simulink model "buoy_detector"  (Simulink 7.6)
settings: Solver=FixedStepDiscrete  StartTime=0.0  StopTime=0  FixedStep=1/30  RelTol=1e-3
values from neighbouring files (symbols this model uses):
  Buoy_Count_Max = 50    [VisionConstants.m]
  Buoy_Count_Min = 3    [VisionConstants.m]
  Buoy_Max_Eccentricity = 1.2    [VisionConstants.m]
  Buoy_Max_Extent = 0.9    [VisionConstants.m]
  Buoy_Min_Eccentricity = 0    [VisionConstants.m]
  Buoy_Min_Extent = 0.1    [VisionConstants.m]
  Iter_Segment_Thresh = 60    [VisionConstants.m]
undefined symbols (not defined in the file or in its folder): Rec, SDTV
libraries: vipgeotforms x3, vipconversions x1
settings Model: Creator=auvt  LastModifiedBy=Administrator
settings RTWCC: TargetLang=C++

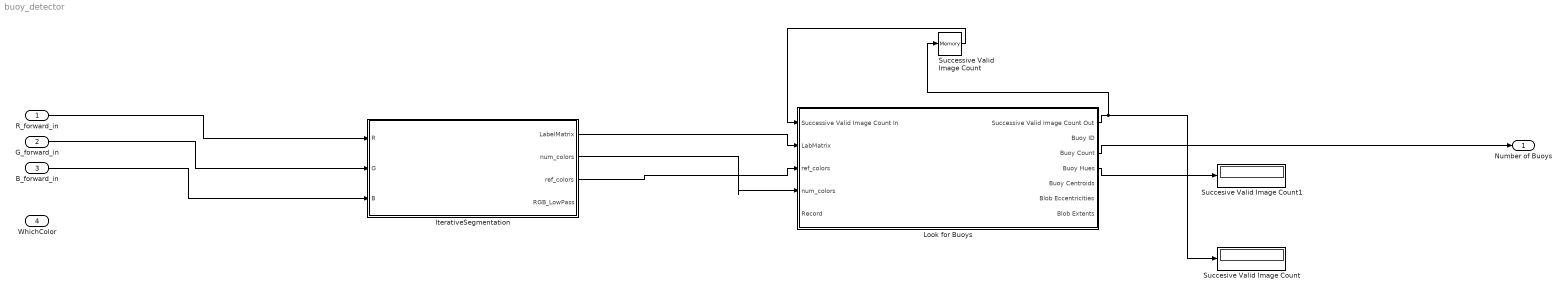
== system buoy_detector ==
  R_forward_in : Inport  PortDimensions=Forward_Camera_Dimensions
  G_forward_in : Inport  Port=2  PortDimensions=Forward_Camera_Dimensions
  B_forward_in : Inport  Port=3  PortDimensions=Forward_Camera_Dimensions
  WhichColor : Inport  Port=4
  IterativeSegmentation : Subsystem
      settings: UndoDeleteFcn=Stateflow.SLINSF.SimulinkMan.restorePreDeleteFcn  PreDeleteFcn=Stateflow.SLINSF.SimulinkMan.removePreDeleteFcn
  Look for Buoys : Subsystem
      settings: UndoDeleteFcn=Stateflow.SLINSF.SimulinkMan.restorePreDeleteFcn  PreDeleteFcn=Stateflow.SLINSF.SimulinkMan.removePreDeleteFcn
  Succesive Valid Image Count : Display
  Succesive Valid Image Count1 : Display
  Successive Valid Image Count : Memory
  Number of Buoys : Outport
  wires:
  IterativeSegmentation/1(LabelMatrix) -> Look for Buoys/2(LabMatrix)
  IterativeSegmentation/3(ref_colors) -> Look for Buoys/3(ref_colors)
  IterativeSegmentation/2(num_colors) -> Look for Buoys/4(num_colors)
  Look for Buoys/3(Buoy Count) -> Number of Buoys/1
  Look for Buoys/1(Successive Valid Image Count Out) -> Succesive Valid Image Count/1, Successive Valid Image Count/1
  Look for Buoys/4(Buoy Hues) -> Succesive Valid Image Count1/1
  Successive Valid Image Count/1 -> Look for Buoys/1(Successive Valid Image Count In)
  R_forward_in/1 -> IterativeSegmentation/1(R)
  G_forward_in/1 -> IterativeSegmentation/2(G)
  B_forward_in/1 -> IterativeSegmentation/3(B)

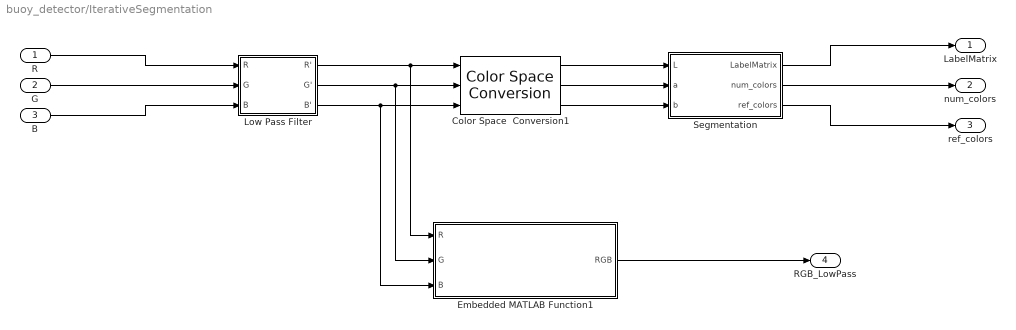
== system buoy_detector/IterativeSegmentation ==
  R : Inport
  G : Inport  Port=2
  B : Inport  Port=3
  Color Space  Conversion1 : vipconversions/Color Space  Conversion  conversion=Obsolete  conversionActive=sR'G'B' to L*a*b*  wp_str=D50  rec=Rec. 601 (SDTV)  sys=1125/60/2:1  imagePorts=Separate color signals
  Embedded MATLAB Function1 : Stateflow chart  TreatAsAtomicUnit=on
  Low Pass Filter : Subsystem
  Segmentation : Subsystem
  LabelMatrix : Outport
  num_colors : Outport  Port=2
  ref_colors : Outport  Port=3
  RGB_LowPass : Outport  Port=4
  wires:
  Segmentation/3(ref_colors) -> ref_colors/1
  Segmentation/2(num_colors) -> num_colors/1
  Segmentation/1(LabelMatrix) -> LabelMatrix/1
  Low Pass Filter/3(B') -> Color Space  Conversion1/3, Embedded MATLAB Function1/3(B)
  Low Pass Filter/2(G') -> Color Space  Conversion1/2, Embedded MATLAB Function1/2(G)
  Low Pass Filter/1(R') -> Color Space  Conversion1/1, Embedded MATLAB Function1/1(R)
  Color Space  Conversion1/3 -> Segmentation/3(b)
  Color Space  Conversion1/2 -> Segmentation/2(a)
  Color Space  Conversion1/1 -> Segmentation/1(L)
  Embedded MATLAB Function1/1(RGB) -> RGB_LowPass/1
  R/1 -> Low Pass Filter/1(R)
  G/1 -> Low Pass Filter/2(G)
  B/1 -> Low Pass Filter/3(B)

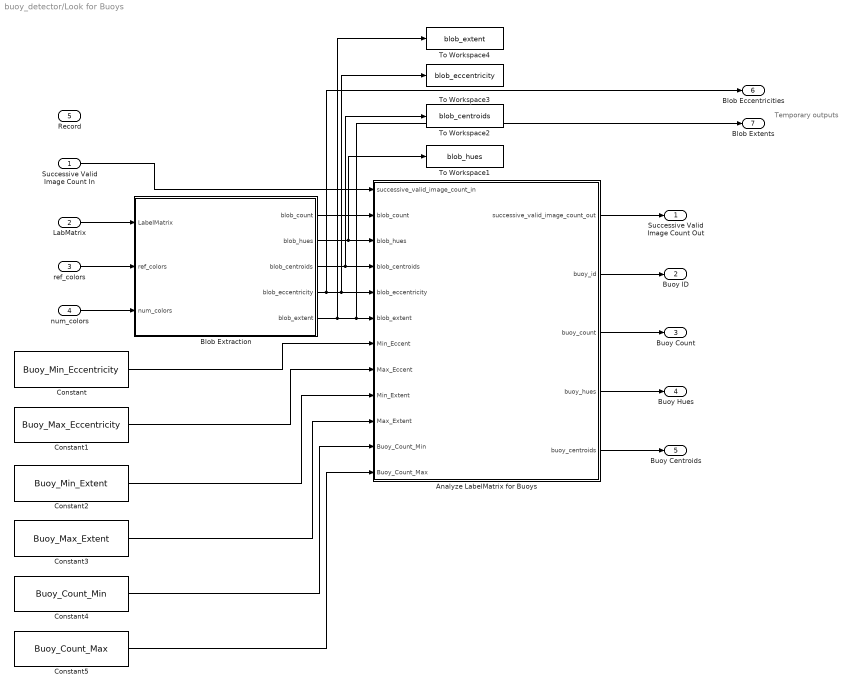
== system buoy_detector/Look for Buoys ==
  note: Temporary outputs
  Successive Valid Image Count In : Inport
  LabMatrix : Inport  Port=2
  ref_colors : Inport  Port=3
  num_colors : Inport  Port=4
  Record : Inport  Port=5
  Analyze LabelMatrix for Buoys : Stateflow chart  TreatAsAtomicUnit=on
  Blob Extraction : Stateflow chart  TreatAsAtomicUnit=on
  Constant : Constant  Value=Buoy_Min_Eccentricity  SampleTime=-1
  Constant1 : Constant  Value=Buoy_Max_Eccentricity  SampleTime=-1
  Constant2 : Constant  Value=Buoy_Min_Extent  SampleTime=-1
  Constant3 : Constant  Value=Buoy_Max_Extent  SampleTime=-1
  Constant4 : Constant  Value=Buoy_Count_Min  SampleTime=-1
  Constant5 : Constant  Value=Buoy_Count_Max  SampleTime=-1
  To Workspace1 : ToWorkspace  VariableName=blob_hues  SampleTime=-1  SaveFormat=Array
  To Workspace2 : ToWorkspace  VariableName=blob_centroids  SampleTime=-1  SaveFormat=Array
  To Workspace3 : ToWorkspace  VariableName=blob_eccentricity  SampleTime=-1  SaveFormat=Array
  To Workspace4 : ToWorkspace  VariableName=blob_extent  SampleTime=-1  SaveFormat=Array
  Successive Valid Image Count Out : Outport
  Buoy ID : Outport  Port=2
  Buoy Count : Outport  Port=3
  Buoy Hues : Outport  Port=4
  Buoy Centroids : Outport  Port=5
  Blob Eccentricities : Outport  Port=6
  Blob Extents : Outport  Port=7
  wires:
  num_colors/1 -> Blob Extraction/3(num_colors)
  LabMatrix/1 -> Blob Extraction/1(LabelMatrix)
  Blob Extraction/1(blob_count) -> Analyze LabelMatrix for Buoys/2(blob_count)
  Blob Extraction/2(blob_hues) -> Analyze LabelMatrix for Buoys/3(blob_hues), To Workspace1/1
  Blob Extraction/3(blob_centroids) -> Analyze LabelMatrix for Buoys/4(blob_centroids), To Workspace2/1
  Blob Extraction/4(blob_eccentricity) -> Analyze LabelMatrix for Buoys/5(blob_eccentricity), To Workspace3/1, Blob Eccentricities/1
  Blob Extraction/5(blob_extent) -> To Workspace4/1, Analyze LabelMatrix for Buoys/6(blob_extent), Blob Extents/1
  Constant/1 -> Analyze LabelMatrix for Buoys/7(Min_Eccent)
  Constant1/1 -> Analyze LabelMatrix for Buoys/8(Max_Eccent)
  Constant2/1 -> Analyze LabelMatrix for Buoys/9(Min_Extent)
  Constant3/1 -> Analyze LabelMatrix for Buoys/10(Max_Extent)
  Constant4/1 -> Analyze LabelMatrix for Buoys/11(Buoy_Count_Min)
  Constant5/1 -> Analyze LabelMatrix for Buoys/12(Buoy_Count_Max)
  Analyze LabelMatrix for Buoys/1(successive_valid_image_count_out) -> Successive Valid Image Count Out/1
  Analyze LabelMatrix for Buoys/3(buoy_count) -> Buoy Count/1
  Analyze LabelMatrix for Buoys/4(buoy_hues) -> Buoy Hues/1
  Analyze LabelMatrix for Buoys/5(buoy_centroids) -> Buoy Centroids/1
  Successive Valid Image Count In/1 -> Analyze LabelMatrix for Buoys/1(successive_valid_image_count_in)
  ref_colors/1 -> Blob Extraction/2(ref_colors)
  Analyze LabelMatrix for Buoys/2(buoy_id) -> Buoy ID/1

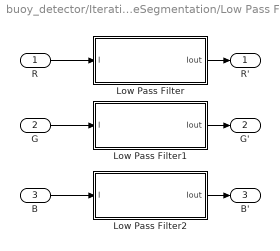
== system buoy_detector/IterativeSegmentation/Low Pass Filter ==
  R : Inport
  G : Inport  Port=2
  B : Inport  Port=3
  Low Pass Filter : Stateflow chart  TreatAsAtomicUnit=on
  Low Pass Filter1 : Stateflow chart  TreatAsAtomicUnit=on
  Low Pass Filter2 : Stateflow chart  TreatAsAtomicUnit=on
  R' : Outport
  G' : Outport  Port=2
  B' : Outport  Port=3
  wires:
  Low Pass Filter/1(Iout) -> R'/1
  Low Pass Filter2/1(Iout) -> B'/1
  Low Pass Filter1/1(Iout) -> G'/1
  B/1 -> Low Pass Filter2/1(I)
  G/1 -> Low Pass Filter1/1(I)
  R/1 -> Low Pass Filter/1(I)

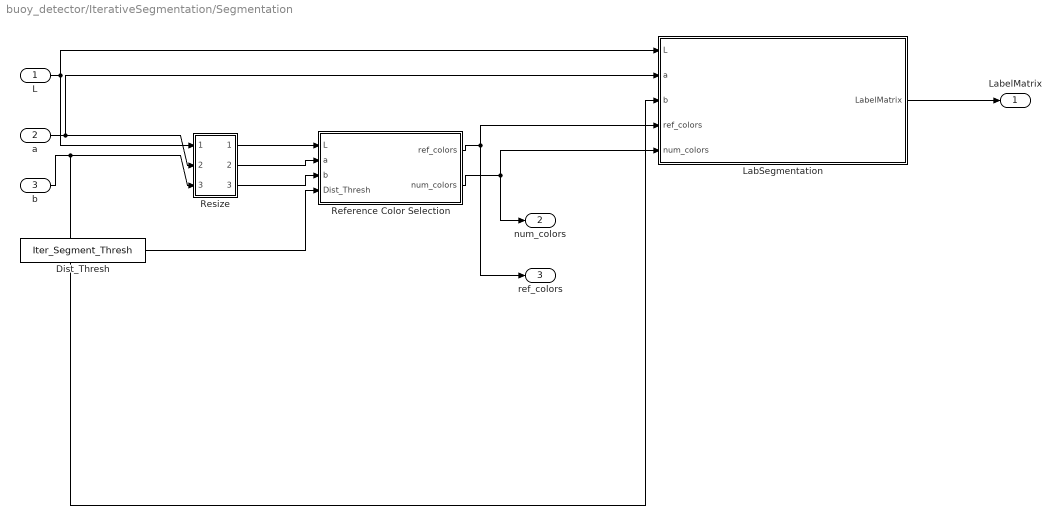
== system buoy_detector/IterativeSegmentation/Segmentation ==
  L : Inport
  a : Inport  Port=2
  b : Inport  Port=3
  Dist_Thresh : Constant  Value=Iter_Segment_Thresh  SampleTime=-1
  LabSegmentation : Stateflow chart  TreatAsAtomicUnit=on
  Reference Color Selection : Stateflow chart  TreatAsAtomicUnit=on
  Resize : Subsystem
  LabelMatrix : Outport
  num_colors : Outport  Port=2
  ref_colors : Outport  Port=3
  wires:
  Dist_Thresh/1 -> Reference Color Selection/4(Dist_Thresh)
  LabSegmentation/1(LabelMatrix) -> LabelMatrix/1
  Reference Color Selection/2(num_colors) -> LabSegmentation/5(num_colors), num_colors/1
  Reference Color Selection/1(ref_colors) -> ref_colors/1, LabSegmentation/4(ref_colors)
  Resize/3(Out3) -> Reference Color Selection/3(b)
  Resize/2(Out2) -> Reference Color Selection/2(a)
  Resize/1(Out1) -> Reference Color Selection/1(L)
  b/1 -> LabSegmentation/3(b), Resize/3(In3)
  a/1 -> LabSegmentation/2(a), Resize/2(In2)
  L/1 -> LabSegmentation/1(L), Resize/1(In1)

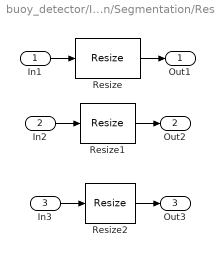
== system buoy_detector/IterativeSegmentation/Segmentation/Resize ==
  In1 : Inport
  In2 : Inport  Port=2
  In3 : Inport  Port=3
  Resize : vipgeotforms/Resize  DialogController=vipDDGCreate  DialogControllerArgs=DataTag0  specify=Number of output rows and columns  rfactor=[]  outCols=25  outRows=25  outRowsCols=[60 80]  interp_method=Bilinear  antialias=on  useROI=off  roiFlag=off  prodOutputMode=Binary point scaling  prodOutputWordLength=32  prodOutputFracLength=10  roundingMode=Nearest  overflowMode=on
  Resize1 : vipgeotforms/Resize  DialogController=vipDDGCreate  DialogControllerArgs=DataTag1  specify=Number of output rows and columns  rfactor=[200 150]  outCols=25  outRows=25  outRowsCols=[60 80]  interp_method=Bilinear  antialias=on  useROI=off  roiFlag=off  prodOutputMode=Binary point scaling  prodOutputWordLength=32  prodOutputFracLength=10  roundingMode=Nearest  overflowMode=on
  Resize2 : vipgeotforms/Resize  DialogController=vipDDGCreate  DialogControllerArgs=DataTag2  specify=Number of output rows and columns  rfactor=[200 150]  outCols=25  outRows=25  outRowsCols=[60 80]  interp_method=Bilinear  antialias=on  useROI=off  roiFlag=off  prodOutputMode=Binary point scaling  prodOutputWordLength=32  prodOutputFracLength=10  roundingMode=Nearest  overflowMode=on
  Out1 : Outport
  Out2 : Outport  Port=2
  Out3 : Outport  Port=3
  wires:
  Resize2/1 -> Out3/1
  In3/1 -> Resize2/1
  Resize1/1 -> Out2/1
  In2/1 -> Resize1/1
  Resize/1 -> Out1/1
  In1/1 -> Resize/1

== matlab function Look for Buoys/Blob Extraction ==
  data: blob_count output double; blob_hues output double; blob_centroids output double; LabelMatrix input double; ref_colors input double; blob_eccentricity output double; num_colors input double; blob_extent output double
function [blob_count, blob_hues, blob_centroids, blob_eccentricity, blob_extent] = GetBlobInfo(LabelMatrix, ref_colors, num_colors)
% This function will determine the characteristics of the blobs in an image
% given a label matrix defining the different binary images contained in a
% that label matrix
%
% Input
%   LabelMatrix = 2-D matrix of integer values, each of which represents a
%     color; location in matrix corresponds to pixel location in image
%   num_colors = integer number of colors present in LabelMatrix
%
% Output
%   blob_count = integer number of blobs in image
%   blob_hues = Nx1 vector of hues of blobs in image
%   blob_centroids = Nx2 matrix of x-y pairs of blob centroid locations
%   blob_eccentricity = Nx1 vector of blob eccentricites
%   blob_extent = Nx1 vector of blob extents


% Initialize
[rows, cols] = size(LabelMatrix);
LogicMatrix = false(rows,cols);

max_num_blobs = 50;
min_blob_area = 5;

blob_hues = double(zeros(max_num_blobs,3));
blob_centroids = double(zeros(max_num_blobs,2));
blob_eccentricity = double(zeros(max_num_blobs,1));
blob_extent = double(zeros(max_num_blobs,1));

blob_count = double(0);%uint8(0);

% Input hblob, a matrix containing [Area, blob_centroids, Eccentricity] for each
% identified blob
persistent hblob
if isempty(hblob)
    hblob = video.BlobAnalysis('AreaOutputPort',false,'BoundingBoxOutputPort',false,...
        'CentroidOutputPort',true,'EccentricityOutputPort',true,'ExtentOutputPort',true,...
        'NumBlobsOutputPort',true,'MinimumBlobAreaSource','Property',...
        'MinimumBlobArea', min_blob_area);
end

%% Calculate geometric information about the blobs
%
% LogicMatrix is a binary version of LabelMatrix, with ones at all
%   locations for which color values are k, and zeros everywhere else
for k = 1:num_colors
    for i = 1:rows
        for j = 1:cols
            if(LabelMatrix(i,j) ~= k)
                LogicMatrix(i,j) = false;
            else
                LogicMatrix(i,j) = true;
            end
        end
    end
    [TCentroid,TEccent,TExtent,TNumBlobs] = step(hblob,LogicMatrix);
    
    if(blob_count+TNumBlobs < max_num_blobs)
        for i = 1:TNumBlobs
            
            blob_centroids(blob_count+i,1) = TCentroid(1,i);
            blob_centroids(blob_count+i,2) = TCentroid(2,i);
            blob_eccentricity(blob_count+i) = TEccent(i);
            blob_extent(blob_count+i) = TExtent(i);
            
            ii = round(blob_centroids(blob_count+i,1));
            jj = round(blob_centroids(blob_count+i,2));
            blob_hues(blob_count+i,1) = ref_colors( LabelMatrix(ii,jj) );
            
        end
        blob_count = blob_count + 1;%TNumBlobs;
    end
end

return

== matlab function Look for Buoys/Analyze LabelMatrix for Buoys ==
  data: successive_valid_image_count_in input double; successive_valid_image_count_out output double; buoy_id output double; blob_count input double; blob_hues input double; blob_centroids input double; buoy_count output double; buoy_hues output double; buoy_centroids output double; blob_eccentricity input double; blob_extent input double; Min_Eccent input double; Max_Eccent input double; Min_Extent input double; Max_Extent input double; Buoy_Count_Min input double; Buoy_Count_Max input double
function [successive_valid_image_count_out, buoy_id, buoy_count, buoy_hues, buoy_centroids] = Buoy_Extraction(successive_valid_image_count_in, blob_count, blob_hues, blob_centroids, blob_eccentricity, blob_extent, Min_Eccent, Max_Eccent, Min_Extent, Max_Extent, Buoy_Count_Min, Buoy_Count_Max)
% This function takes in vectors representing blobs present in the image,
%   and returns information about how many and what kind of buoys are
%   present.
%
% Input
%   blob_count = integer number of blobs in image
%   blob_hues = Nx1 vector of hues of blobs in image
%   blob_centroids = Nx2 matrix of x-y pairs of blob centroid locations
%   blob_eccentricity = Nx1 vector of blob eccentricites
%   blob_extent = Nx1 vector of blob extents
%
%   Buoy_Count_Min = integer; minimum number of buoys searched for in an
%     image (mission/controls needs requires this option)
%   Buoy_Count_Max = maximum number of buoys allowed per image; arbitrary
%     limit
%   Min_Hue,Max_Hue = Nx1 limits on valid buoy hues; hue is between 0 and 1
%   Min_Eccent,Max_Eccent = scalar limits on buoy eccentricity
%   Min_Extent,Max_Extent = scalar limits on buoy extent
%
% Output
%   successive_valid_image_count = integer value of the number of times an
%     image with more than Min_Num_Buoys is processed; persistant between
%     function calls, so that the number of successive images containing
%     at least Min_Num_Buoys buoys is tracked
%   buoy_count = integer number of buoys in image
%   buoy_hues = Nx1 vector of buoy colors
%   buoy_centroids = Nx2 matrix of x-y pairs of buoy centroid locations


% Initialize
%persistent successive_valid_image_count;
buoy_count = double(0);

%debug
%successive_valid_image_count = 0;
Buoy_Count_Max = 50;


%/debug
buoy_hues = double(zeros(Buoy_Count_Max,1));
buoy_centroids = double(-500.*ones(Buoy_Count_Max,2));  % Initialize to points clearly not located in image

buoy_id = double(-1.*ones(Buoy_Count_Max,1));
Buoy_Hue_HalfRange = 10;
Buoy1_Hue = 30;
Buoy2_Hue = 80;
Buoy3_Hue = 15;

% Loop through blobs, and analyze and extract buoy information
for i = 1:blob_count
    
    % Convert Lab to XYZ
%    R = buoy_hues(i);
%    G = buoy_hues(i);
%    B = buoy_hues(i);
    
    L = blob_hues(:,1); %refcolors(LabelMatrix(1,1,1));
    a = blob_hues(:,2);
    b = blob_hues(:,3);
    
    var_Y = L./10;
    var_X = ( a./17.5 ).*( L./10 );
    var_Z = ( b./7 ).*( L./10 );
    
    Y = var_Y.^2;
    X = ( var_X + Y )./1.02;
    Z = -( var_Z - Y )./0.847;
    
    % Convert XYZ to RGB
    var_X = X./100;        %X from 0 to  95.047      (Observer = 2 degrees, Illuminant = D65)
    var_Y = Y./100;        %Y from 0 to 100.000
    var_Z = Z./100;        %Z from 0 to 108.883
    
    var_R = var_X.*3.2406 + var_Y.*(-1.5372) + var_Z.* -0.4986;
    var_G = var_X .* -0.9689 + var_Y .*  1.8758 + var_Z.*  0.0415;
    var_B = var_X .*  0.0557 + var_Y .* -0.2040 + var_Z .*  1.0570;
    
    var_R = ( var_R > 0.0031308 ).*( 1.055.*( var_R.^( 1./2.4 ) ) - 0.055 ) + ( var_R <= 0.0031308 ).*(12.92.*var_R);
    var_G = ( var_G > 0.0031308 ).*( 1.055.*( var_G.^( 1./2.4 ) ) - 0.055 ) + ( var_G <= 0.0031308 ).*( var_G <= 12.92.*var_G );
    var_B = ( var_B > 0.0031308 ).*( 1.055 .* ( var_B .^ ( 1 ./ 2.4 ) ) - 0.055 ) + ( var_B <= 0.0031308 ).*( 12.92 .* var_B );
    
    R = var_R .* 255;
    G = var_G .* 255;
    B = var_B .* 255;
    
    % Convert RGB to HSV
    var_R = ( R ./ 255 );  % RGB from 0 to 255
    var_G = ( G ./ 255 );
    var_B = ( B ./ 255 );
    
    var_Min = min( [var_R, var_G, var_B], [], 2 );  % Min. value of RGB
    var_Max = max( [var_R, var_G, var_B], [], 2 );  % Max. value of RGB
    del_Max = var_Max - var_Min;  % Delta RGB value
    
    V = var_Max;
    
%    H = (del_Max != 0).*(  );
%    S = (del_Max != 0).*( del_Max./var_Max );
    if ( max(abs(del_Max == 0)) );  % This is a gray, no chroma...
        H = zeros(size(var_R));  % HSV results from 0 to 1
        S = zeros(size(var_R));
    else  % Chromatic data...
        
        S = del_Max ./ var_Max;
        
        del_R = ( ( ( var_Max - var_R ) ./ 6 ) + ( del_Max ./ 2 ) ) ./ del_Max;
        del_G = ( ( ( var_Max - var_G ) ./ 6 ) + ( del_Max ./ 2 ) ) ./ del_Max;
        del_B = ( ( ( var_Max - var_B ) ./ 6 ) + ( del_Max ./ 2 ) ) ./ del_Max;
        
        
        H = ( var_R == var_Max ).*( del_B - del_G ) + ( var_G == var_Max ).*( ( 1 ./ 3 ) + del_R - del_B ) + ( var_B == var_Max ).*( ( 2 ./ 3 ) + del_G - del_R );
        H = ( H < 0 ).*( H + 1 ) + ( H > 1 ).*( H - 1 );
        
        
%{        
        if( var_R == var_Max )
            H = del_B - del_G;
        elseif( var_G == var_Max )
            H = ( 1 ./ 3 ) + del_R - del_B;
        elseif( var_B == var_Max )
            H = ( 2 ./ 3 ) + del_G - del_R;
        else
            H = 0;
        end
        
        if( H < 0 )
            H = H + 1;
        end
        if( H > 1 )
            H = H - 1;
        end
%}        
    end
    
    
    
    
    
    
    
    
    
    % Store buoy information if blob conditions are met
    %   Conditions: 1) Blob eccentricity is within specified range
    %               2) Blob extent is within specified range
    %               3) Blob hue is within specified range for several buoy
    %                 types
    if( (blob_eccentricity(i)>=Min_Eccent) && (blob_eccentricity(i)<=Max_Eccent) && (blob_extent(i)>=Min_Extent) && (blob_extent(i)<=Max_Extent) )
        
        %if( (blob_hues(i)>=Buoy1_Hue-Buoy_Hue_HalfRange) && (blob_hues(i)<=Buoy1_Hue+Buoy_Hue_HalfRange) )
            buoy_count = buoy_count + 1;
            buoy_hues(buoy_count) = blob_hues(i);
            buoy_id(buoy_count) = 1;
            buoy_centroids(buoy_count,1) = blob_centroids(i,1);
            buoy_centroids(buoy_count,2) = blob_centroids(i,2);
        %end
        if( (blob_hues(i)>=Buoy2_Hue-Buoy_Hue_HalfRange) && (blob_hues(i)<=Buoy2_Hue+Buoy_Hue_HalfRange) )
            buoy_count = buoy_count + 1;
            buoy_hues(buoy_count) = blob_hues(i);
            buoy_id(buoy_count) = 2;
            buoy_centroids(buoy_count,1) = blob_centroids(i,1);
            buoy_centroids(buoy_count,2) = blob_centroids(i,2);
        end
        if( (blob_hues(i)>=Buoy3_Hue-Buoy_Hue_HalfRange) && (blob_hues(i)<=Buoy3_Hue+Buoy_Hue_HalfRange) )
            buoy_count = buoy_count + 1;
            buoy_hues(buoy_count) = blob_hues(i);
            buoy_id(buoy_count) = 3;
            buoy_centroids(buoy_count,1) = blob_centroids(i,1);
            buoy_centroids(buoy_count,2) = blob_centroids(i,2);
        end
    end
    
end

if( buoy_count >= Buoy_Count_Min )
    successive_valid_image_count_out = double(successive_valid_image_count_in + 1);
else
    successive_valid_image_count_out = double(0);
end


% Resize output arrays
%buoy_hues = buoy_hues(1:buoy_count);
%buoy_centroids = buoy_centroids(1:buoy_count,:);
%buoy_id = ;

return

== matlab function IterativeSegmentation/Embedded MATLAB Function1 ==
  data: R input double; RGB output double; G input double; B input double
function RGB = SeparatetoSingleSignals(R,G,B)
% This function combines the separate color signals into a single 3-D signal

[rows, cols] = size(R);

RGB = zeros(rows,cols,3);

for i = 1:rows
    for j = 1:cols
        RGB(i,j,1) = R(i,j);
        RGB(i,j,2) = G(i,j);
        RGB(i,j,3) = B(i,j);
    end
end

return

== matlab function IterativeSegmentation/Low Pass Filter/Low Pass Filter ==
  data: I input double; Iout output double
function Iout = GaussianBlurr(I)
% This function calculates the gaussian blur of an intensity image

sigma = sqrt(2);

Grows = 3;    % Gaussian matrix rows
Gcols = 3;    % Gaussian matrix columns

[Irows Icols] = size(I);

Iout = double(zeros(Irows,Icols));

Trows = Irows - Grows + 1;
Tcols = Icols - Gcols + 1;
Itemp = double(zeros(Trows,Tcols));

G = zeros(Grows,Gcols);

FirstRow = ceil(-Grows/2);
LastRow = floor(Grows/2);
FirstCol = ceil(-Gcols/2);
LastCol = floor(Gcols/2);
Gsum = 0;
for i=FirstRow:LastRow
    for j = FirstCol:LastCol
        G(i-FirstRow+1,j-FirstCol+1) = exp(-(j*j+i*i)/(2*sigma*sigma));
        Gsum = Gsum + G(i-FirstRow+1,j-FirstCol+1);
    end
end

G = G./Gsum;

Itemp = conv2(double(I),double(G),'valid');

% reflect boundaries to keep image the same size
% top
Iout((1:LastRow),(LastCol+1:Icols-LastCol)) = Itemp((1:LastRow),(1:Tcols));
% bottom
Iout((Irows-LastRow+1:Irows),(LastCol+1:Icols-LastCol)) = Itemp((Trows-LastRow+1:Trows),(1:Tcols));
% left
Iout((1+LastRow:Irows-LastRow),(1:LastCol)) = Itemp((1:Trows),(1:LastCol));
% right
Iout((1+LastRow:Irows-LastRow),(Icols-LastCol+1:Icols)) = Itemp((1:Trows),(Tcols-LastCol+1:Tcols));
% center
Iout((1+LastRow:Irows-LastRow),(1+LastCol:Icols-LastCol)) = Itemp;
% top left corner
Iout(1:LastRow,1:LastCol) = Itemp(1:LastRow,1:LastCol);
% top right corner
Iout(1:LastRow,Icols-LastCol:Icols) = Itemp(1:LastRow,Tcols-LastCol:Tcols);
% bottom left corner
Iout(Irows-LastRow:Irows,1:LastCol) = Itemp(Trows-LastRow:Trows,1:LastCol);
% bottom right corner
Iout(Irows-LastRow:Irows,Icols-LastCol:Icols) = Itemp(Trows-LastRow:Trows,Tcols-LastCol:Tcols);

return

== matlab function IterativeSegmentation/Low Pass Filter/Low Pass Filter1 ==
  data: I input double; Iout output double
function Iout = GaussianBlurr(I)
% This function calculates the gaussian blur of an intensity image

sigma = sqrt(2);

Grows = 3;    % Gaussian matrix rows
Gcols = 3;    % Gaussian matrix columns

[Irows Icols] = size(I);

Iout = double(zeros(Irows,Icols));

Trows = Irows - Grows + 1;
Tcols = Icols - Gcols + 1;
Itemp = double(zeros(Trows,Tcols));

G = zeros(Grows,Gcols);

FirstRow = ceil(-Grows/2);
LastRow = floor(Grows/2);
FirstCol = ceil(-Gcols/2);
LastCol = floor(Gcols/2);
Gsum = 0;
for i=FirstRow:LastRow
    for j = FirstCol:LastCol
        G(i-FirstRow+1,j-FirstCol+1) = exp(-(j*j+i*i)/(2*sigma*sigma));
        Gsum = Gsum + G(i-FirstRow+1,j-FirstCol+1);
    end
end

G = G./Gsum;

Itemp = conv2(double(I),double(G),'valid');

% reflect boundaries to keep image the same size
% top
Iout((1:LastRow),(LastCol+1:Icols-LastCol)) = Itemp((1:LastRow),(1:Tcols));
% bottom
Iout((Irows-LastRow+1:Irows),(LastCol+1:Icols-LastCol)) = Itemp((Trows-LastRow+1:Trows),(1:Tcols));
% left
Iout((1+LastRow:Irows-LastRow),(1:LastCol)) = Itemp((1:Trows),(1:LastCol));
% right
Iout((1+LastRow:Irows-LastRow),(Icols-LastCol+1:Icols)) = Itemp((1:Trows),(Tcols-LastCol+1:Tcols));
% center
Iout((1+LastRow:Irows-LastRow),(1+LastCol:Icols-LastCol)) = Itemp;
% top left corner
Iout(1:LastRow,1:LastCol) = Itemp(1:LastRow,1:LastCol);
% top right corner
Iout(1:LastRow,Icols-LastCol:Icols) = Itemp(1:LastRow,Tcols-LastCol:Tcols);
% bottom left corner
Iout(Irows-LastRow:Irows,1:LastCol) = Itemp(Trows-LastRow:Trows,1:LastCol);
% bottom right corner
Iout(Irows-LastRow:Irows,Icols-LastCol:Icols) = Itemp(Trows-LastRow:Trows,Tcols-LastCol:Tcols);

return

== matlab function IterativeSegmentation/Low Pass Filter/Low Pass Filter2 ==
  data: I input double; Iout output double
function Iout = GaussianBlurr(I)
% This function calculates the gaussian blur of an intensity image

sigma = sqrt(2);

Grows = 3;    % Gaussian matrix rows
Gcols = 3;    % Gaussian matrix columns

[Irows Icols] = size(I);

Iout = double(zeros(Irows,Icols));

Trows = Irows - Grows + 1;
Tcols = Icols - Gcols + 1;
Itemp = double(zeros(Trows,Tcols));

G = zeros(Grows,Gcols);

FirstRow = ceil(-Grows/2);
LastRow = floor(Grows/2);
FirstCol = ceil(-Gcols/2);
LastCol = floor(Gcols/2);
Gsum = 0;
for i=FirstRow:LastRow
    for j = FirstCol:LastCol
        G(i-FirstRow+1,j-FirstCol+1) = exp(-(j*j+i*i)/(2*sigma*sigma));
        Gsum = Gsum + G(i-FirstRow+1,j-FirstCol+1);
    end
end

G = G./Gsum;

Itemp = conv2(double(I),double(G),'valid');

% reflect boundaries to keep image the same size
% top
Iout((1:LastRow),(LastCol+1:Icols-LastCol)) = Itemp((1:LastRow),(1:Tcols));
% bottom
Iout((Irows-LastRow+1:Irows),(LastCol+1:Icols-LastCol)) = Itemp((Trows-LastRow+1:Trows),(1:Tcols));
% left
Iout((1+LastRow:Irows-LastRow),(1:LastCol)) = Itemp((1:Trows),(1:LastCol));
% right
Iout((1+LastRow:Irows-LastRow),(Icols-LastCol+1:Icols)) = Itemp((1:Trows),(Tcols-LastCol+1:Tcols));
% center
Iout((1+LastRow:Irows-LastRow),(1+LastCol:Icols-LastCol)) = Itemp;
% top left corner
Iout(1:LastRow,1:LastCol) = Itemp(1:LastRow,1:LastCol);
% top right corner
Iout(1:LastRow,Icols-LastCol:Icols) = Itemp(1:LastRow,Tcols-LastCol:Tcols);
% bottom left corner
Iout(Irows-LastRow:Irows,1:LastCol) = Itemp(Trows-LastRow:Trows,1:LastCol);
% bottom right corner
Iout(Irows-LastRow:Irows,Icols-LastCol:Icols) = Itemp(Trows-LastRow:Trows,Tcols-LastCol:Tcols);

return

== matlab function IterativeSegmentation/Segmentation/LabSegmentation ==
  data: L input double; LabelMatrix output double; a input double; b input double; ref_colors input double; num_colors input double
function LabelMatrix  = LabSegmentation(L,a,b,ref_colors,num_colors)
% This function generates the label matrix

[rows cols] = size(L);

Lout = zeros(rows,cols);
aout = zeros(rows,cols);
bout = zeros(rows,cols);

LabelMatrix = zeros(rows,cols);

for i = 1:rows
    for j = 1:cols
        min_dist = 1000;
        index = 1;
        for k = 1:num_colors
            dist = sqrt((ref_colors(k,1) - L(i,j))^2 + (ref_colors(k,2) - a(i,j))^2 + (ref_colors(k,3) - b(i,j))^2);
            if(dist < min_dist)
                min_dist = double(dist);
                index = k;
            end
        end
        LabelMatrix(i,j) = index;
    end
end

for i = 1:rows
    for j = 1:cols
        Lout(i,j) = ref_colors(LabelMatrix(i,j),1);
        aout(i,j) = ref_colors(LabelMatrix(i,j),2);
        bout(i,j) = ref_colors(LabelMatrix(i,j),3);
    end
end

cow = 1;

return

== matlab function IterativeSegmentation/Segmentation/Reference Color Selection ==
  data: L input double; ref_colors output double; a input double; b input double; num_colors output double; Dist_Thresh input double
function [ref_colors, num_colors] = Segmentation(L,a,b,Dist_Thresh)
% This function tries segmentation by adding new reference colors everytime
% a pixel is found with a distance greater than a certain amount from
% every other reference color

[rows cols] = size(L);

Dist_Threshold = Dist_Thresh;% L = 0 to 100, a = -100 to 100, b = -100 to 100
                    % max dist = 300 -> 60/300 is 20%
x = 1;  % coefficients determining distance calculation
y = 1.5;
z = 1.5;

max_num_colors = 50;
ref_colors = zeros(max_num_colors,3);   % At most 50 different reference colors
LabelMatrix = zeros(rows,cols);
num_colors = 1;

center_row = floor(rows/2);
center_col = floor(cols/2);

% Define first reference color to be colr
ref_colors(1,:) = [L(center_row,center_col) a(center_row,center_col) b(center_row,center_col)];

flag = 0;
i = 1;
j = 1;
while(i <= rows)        % perform initial segmentation
    while(i <= rows && flag == 0)
        while(j <= cols && flag == 0)
            k = 1;
            min_dist = 1000;
            index = 1;
            while(k <= num_colors)
                dist = sqrt(x*(ref_colors(k,1) - L(i,j))^2 + y*(ref_colors(k,2) - a(i,j))^2 + z*(ref_colors(k,3) - b(i,j))^2);
                if(min_dist > dist)
                    min_dist = double(dist);
                    index = k;
                end
                k = k + 1;
            end
            if(j == 117)
                cow = 1;
            end
            if(min_dist > Dist_Threshold && num_colors < max_num_colors)
                ref_colors(num_colors+1,:) = [L(i,j) a(i,j) b(i,j)];
                num_colors = num_colors + 1;
                flag = 1;
                i = 0;
                j = 0;
            else
                LabelMatrix(i,j) = index;
            end
            j = j + 1;
        end
        j = 1;
        i = i + 1;
    end
    flag = 0;
end

% Go through image once more to get more accurate values for the different regions
ref_color_L_avg = zeros(50,1);
ref_color_a_avg = zeros(50,1);
ref_color_b_avg = zeros(50,1);
color_count = zeros(50,1);
for i = 1:rows
    for j = 1:cols
        index = LabelMatrix(i,j);
        ref_color_L_avg(index) = ref_color_L_avg(index) + L(i,j);
        ref_color_a_avg(index) = ref_color_a_avg(index) + a(i,j);
        ref_color_b_avg(index) = ref_color_b_avg(index) + b(i,j);
        color_count(index) = color_count(index) + 1;
    end
end
ref_color_L_avg = ref_color_L_avg ./ color_count;
ref_color_a_avg = ref_color_a_avg ./ color_count;
ref_color_b_avg = ref_color_b_avg ./ color_count;

for i = 1:num_colors
    ref_colors(i,1) = ref_color_L_avg(i);
    ref_colors(i,2) = ref_color_a_avg(i);
    ref_colors(i,3) = ref_color_b_avg(i);
end

return
